simulink model "sampleModel367"  (R2021b)
settings: Solver=VariableStepAuto  StartTime=0.0  StopTime=10.0  RelTol=1e-3
undefined symbols (not defined in the file or in its folder): DiscIntNeverNeededParam
libraries: simulink x15, slpidlib x3
settings Model: Creator=user  LastModifiedBy=user

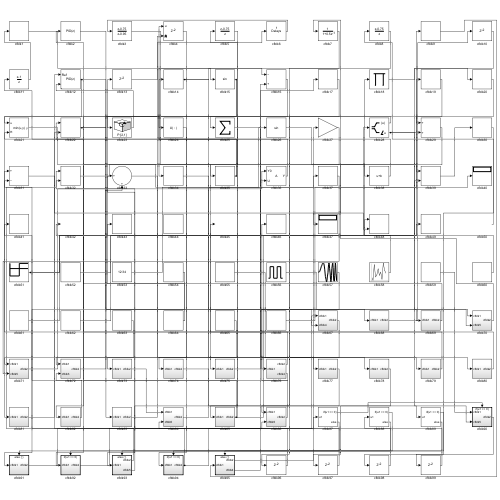
[thumbnail: Simulink's stored preview of the top-level diagram]
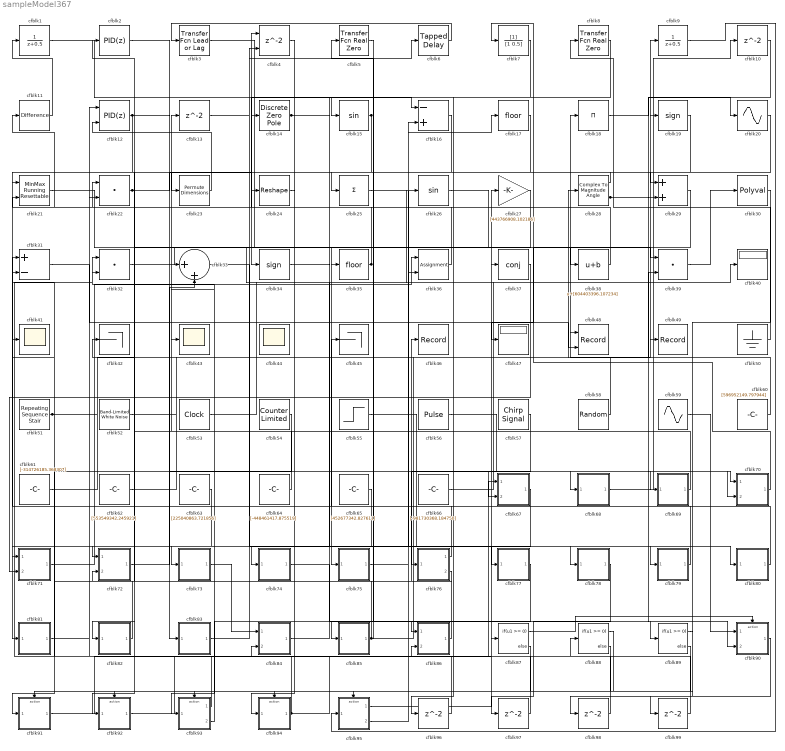
== system sampleModel367 ==
  cfblk1 : DiscreteTransferFcn  SampleTime=1
  cfblk{10,13,96..99} (6 alike) : Delay  SampleTime=1
  cfblk11 : simulink/Discrete/Difference  ICPrevInput=0.0  OutMin=[]  OutMax=[]  OutDataTypeStr=Inherit: Inherit via back propagation  OutDataType=fixdt(1, 16)  OutScaling=2^-10  DoSatur=off
  cfblk12 : slpidlib/PID Controller (2DOF)  Controller=PID  Form=Parallel  TimeDomain=Discrete-time  UseExternalTs=off  SampleTime=1  IntegratorMethod=Forward Euler  FilterMethod=Forward Euler  ControllerParametersSource=internal  P=1  I=1  D=0  UseFilter=on  N=100  b=1  c=1  TunerSelectOption=Transfer Function Based (PID Tuner App)  InitialConditionSource=internal  InitialConditionForIntegrator=0  InitialConditionForFilter=0  DifferentiatorICPrevScaledInput=0  ExternalReset=none  TrackingMode=off  Kt=1  LimitOutput=off  SatLimitsSource=internal  UpperSaturationLimit=inf  LowerSaturationLimit=-inf  LinearizeAsGain=off  AntiWindupMode=none  Kb=1  POutMin=[]  POutMax=[]  IOutMin=[]  IOutMax=[]  DOutMin=[]  DOutMax=[]  NOutMin=[]  NOutMax=[]  bOutMin=[]  bOutMax=[]  cOutMin=[]  cOutMax=[]  SumOutMin=[]  SumOutMax=[]  SaturationOutMin=[]  SaturationOutMax=[]  PParamMin=[]  PParamMax=[]  IParamMin=[]  IParamMax=[]  DParamMin=[]  DParamMax=[]  NParamMin=[]  NParamMax=[]  bParamMin=[]  bParamMax=[]  cParamMin=[]  cParamMax=[]  KbParamMin=[]  KbParamMax=[]  KtParamMin=[]  KtParamMax=[]  KbOutMin=[]  KbOutMax=[]  KtOutMin=[]  KtOutMax=[]  IntegratorOutMin=[]  IntegratorOutMax=[]  FilterOutMin=[]  FilterOutMax=[]  SumI1OutMin=[]  SumI1OutMax=[]  SumI2OutMin=[]  SumI2OutMax=[]  SumI3OutMin=[]  SumI3OutMax=[]  SumI4OutMin=[]  SumI4OutMax=[]  SumDOutMin=[]  SumDOutMax=[]  Sum1OutMin=[]  Sum1OutMax=[]  Sum2OutMin=[]  Sum2OutMax=[]  Sum3OutMin=[]  Sum3OutMax=[]  DifferentiatorOutMin=[]  DifferentiatorOutMax=[]  FilterDiffOutCoefMin=[]  FilterDiffOutCoefMax=[]  ReciprocalOutMin=[]  ReciprocalOutMax=[]  SumDenOutMin=[]  SumDenOutMax=[]  SumNumOutMin=[]  SumNumOutMax=[]  DivideOutMin=[]  DivideOutMax=[]  UdiffTsProdOutMin=[]  UdiffTsProdOutMax=[]  NTsProdOutMin=[]  NTsProdOutMax=[]  UintegralTsProdOutMin=[]  UintegralTsProdOutMax=[]  UngainTsProdOutMin=[]  UngainTsProdOutMax=[]  IntegratorContinuousStateAttributes=''  IntegratorStateMustResolveToSignalObject=off  IntegratorRTWStateStorageClass=Auto  FilterContinuousStateAttributes=''  FilterStateMustResolveToSignalObject=off  FilterRTWStateStorageClass=Auto  ParallelPVariant=InternalParameters  IdealPVariant=Disabled  IVariant=InternalParameters  DVariant=InternalParameters  bVariant=InternalParameters  cVariant=InternalParameters  IntegratorVariant=Discrete  SatVariant=Disabled  AWVariant=Passthrough  PCopyVariant=Disabled  TRVariant=Disabled  FdbkBlocksVariant=Forward  IdealPFdbkVariant=Disabled  SatFdbkVariant=Disabled  DerivativeFilterVariant=ForwardEulerFilter  NVariant=InternalParameters  NCopyVariant=Disabled  FilterICVariant=InternalICsFilter  IntegratorICVariant=InternalICs  ExternalResetVariant=Disabled  TRSumVariant=Passthrough  SumFdbkVariant=Disabled  SumVariant=Sum_PID  TsampFilterVariant=InternalTs  TsampNgainVariant=Passthrough  TsampIntegralVariant=Passthrough  ExternalSaturationOutDataTypeStr=Inherit: Same as second input
      settings: SourceProductBaseCode=SL
  cfblk14 : DiscreteZeroPole  Poles=[0 0.5]  Gain=1
  cfblk15 : Trigonometry
  cfblk16 : Sum  Inputs=-+
  cfblk17 : Rounding
  cfblk18 : Product  Inputs=*
  cfblk19 : Signum
  cfblk2 : slpidlib/PID Controller  Controller=PID  Form=Parallel  TimeDomain=Discrete-time  UseExternalTs=off  SampleTime=1  IntegratorMethod=Forward Euler  FilterMethod=Forward Euler  ControllerParametersSource=internal  P=1  I=1  D=0  UseFilter=on  N=100  TunerSelectOption=Transfer Function Based (PID Tuner App)  InitialConditionSource=internal  InitialConditionForIntegrator=0  InitialConditionForFilter=0  DifferentiatorICPrevScaledInput=0  ExternalReset=none  TrackingMode=off  Kt=1  LimitOutput=off  SatLimitsSource=internal  UpperSaturationLimit=inf  LowerSaturationLimit=-inf  LinearizeAsGain=off  AntiWindupMode=none  Kb=1  POutMin=[]  POutMax=[]  IOutMin=[]  IOutMax=[]  DOutMin=[]  DOutMax=[]  NOutMin=[]  NOutMax=[]  SumOutMin=[]  SumOutMax=[]  SaturationOutMin=[]  SaturationOutMax=[]  PParamMin=[]  PParamMax=[]  IParamMin=[]  IParamMax=[]  DParamMin=[]  DParamMax=[]  NParamMin=[]  NParamMax=[]  KbParamMin=[]  KbParamMax=[]  KtParamMin=[]  KtParamMax=[]  KbOutMin=[]  KbOutMax=[]  KtOutMin=[]  KtOutMax=[]  IntegratorOutMin=[]  IntegratorOutMax=[]  FilterOutMin=[]  FilterOutMax=[]  SumI1OutMin=[]  SumI1OutMax=[]  SumI2OutMin=[]  SumI2OutMax=[]  SumI3OutMin=[]  SumI3OutMax=[]  SumI4OutMin=[]  SumI4OutMax=[]  SumDOutMin=[]  SumDOutMax=[]  DifferentiatorOutMin=[]  DifferentiatorOutMax=[]  FilterDiffOutCoefMin=[]  FilterDiffOutCoefMax=[]  ReciprocalOutMin=[]  ReciprocalOutMax=[]  SumDenOutMin=[]  SumDenOutMax=[]  SumNumOutMin=[]  SumNumOutMax=[]  DivideOutMin=[]  DivideOutMax=[]  UdiffTsProdOutMin=[]  UdiffTsProdOutMax=[]  NTsProdOutMin=[]  NTsProdOutMax=[]  UintegralTsProdOutMin=[]  UintegralTsProdOutMax=[]  UngainTsProdOutMin=[]  UngainTsProdOutMax=[]  IntegratorContinuousStateAttributes=''  IntegratorStateMustResolveToSignalObject=off  IntegratorRTWStateStorageClass=Auto  FilterContinuousStateAttributes=''  FilterStateMustResolveToSignalObject=off  FilterRTWStateStorageClass=Auto  ParallelPVariant=InternalParameters  IdealPVariant=Disabled  IVariant=InternalParameters  DVariant=InternalParameters  IntegratorVariant=Discrete  SatVariant=Disabled  AWVariant=Passthrough  PCopyVariant=Disabled  TRVariant=Disabled  FdbkBlocksVariant=Forward  IdealPFdbkVariant=Disabled  SatFdbkVariant=Disabled  DerivativeFilterVariant=ForwardEulerFilter  NVariant=InternalParameters  NCopyVariant=Disabled  FilterICVariant=InternalICsFilter  IntegratorICVariant=InternalICs  ExternalResetVariant=Disabled  TRSumVariant=Passthrough  SumFdbkVariant=Disabled  SumVariant=Sum_PID  TsampFilterVariant=InternalTs  TsampNgainVariant=Passthrough  TsampIntegralVariant=Passthrough  ExternalSaturationOutDataTypeStr=Inherit: Same as second input
  cfblk20 : Sin  TimeSource=Use external signal  SampleTime=0
  cfblk21 : simulink/Math Operations/MinMax Running Resettable  Function=min  vinit=0.0
  cfblk22 : DotProduct  InputSameDT=on  OutDataTypeStr=Inherit: Inherit via internal rule
  cfblk23 : PermuteDimensions
  cfblk24 : Reshape
  cfblk25 : Sum  Inputs=+
  cfblk26 : Trigonometry
  cfblk27 : Gain  Gain=[443766908.102186]
  cfblk28 : ComplexToMagnitudeAngle
  cfblk29 : Sum
  cfblk3 : simulink/Discrete/Transfer Fcn Lead or Lag  PoleZ=0.95  ZeroZ=0.75  ICPrevOutput=0.0  ICPrevInput=0.0  DoSatur=off
      settings: SourceProductBaseCode=SL
  cfblk30 : Polyval  Coefs=[ +2.081618890e-019, -1.441693666e-014, +4.719686976e-010, -8.536869453e-006, +1.621573104e-001, -8.087801117e+001 ]
  cfblk31 : Sum  Inputs=+-
  cfblk32 : DotProduct  InputSameDT=on  OutDataTypeStr=Inherit: Inherit via internal rule
  cfblk33 : Sum  Inputs=|++
  cfblk34 : Signum
  cfblk35 : Rounding
  cfblk36 : Assignment  DiagnosticForDimensions=Warning  IndexOptions=Index vector (dialog)  Indices=1  OutputSizes=1
  cfblk37 : Math  Operator=conj  SaturateOnIntegerOverflow=on
  cfblk38 : Bias  Bias=[604403396.107234]
  cfblk39 : DotProduct  InputSameDT=on  OutDataTypeStr=Inherit: Inherit via internal rule
  cfblk4 : Delay  ShowEnablePort=on  SampleTime=1
      settings: InputPortMap=u0,e6
  cfblk40 : Display
  cfblk41 : Scope
  cfblk42 : Terminator
  cfblk43 : Scope
  cfblk44 : Scope
      settings: Floating=on
  cfblk45 : Terminator
  cfblk46 : Record  FileSettingsInternal="{\"entries\":[{\"content\":{\"excelSettings\":{\"content\":{},\"type\":\"Streamout.ExcelSettings\"}},\"type\":\"Streamout.FileSettingStorage\",\"uuid\":\"a4817eb2-789e-49c8-9b38-fb696686bad4\"}],\"packageUris\":[\"http://schema.mathworks.com/mf0/streamout_blocks/R2020a\"],\"version\":\"1.0\"}"  SignalsInternal="{\"entries\":[{\"content\":{\"signals\":[{\"content\":{\"blockPath\":[\"sampleModel367/cfblk46\"],\"channel\":[],\"dimensions\":[1],\"domain\":\"sampleModel367/cfblk46\",\"lineColor\":\"#b746ff\",\"plots\":[1],\"port\":1,\"sid\":[\"\"],\"signalID\":15209,\"signalName\":\"cfblk86\"},\"type\":\"RecordBlkView.Signal\",\"uuid\":\"a4bc0313-54ea-4444-9b09-4c15ea739dbc\"}]},\"type\":\"RecordBlkView.InputSignals\",\"uuid\":\"43528cc1-72da-4af5-8b92-5aee9282fc77\"}],\"packageUris\":[\"http://schema.mathworks.com/mf0/streamout_blocks/R2020a\"],\"version\":\"1.0\"}"  VisualizationBindings="{\"sparklinesplugin\":{\"info\":[{\"bindingParametersList\":[],\"subplotID\":1}]}}"
  cfblk47 : Display
  cfblk48 : Record  FileSettingsInternal="{\"entries\":[{\"content\":{\"excelSettings\":{\"content\":{},\"type\":\"Streamout.ExcelSettings\"}},\"type\":\"Streamout.FileSettingStorage\",\"uuid\":\"7f5feb7f-130e-4751-b9c9-40299ce25e98\"}],\"packageUris\":[\"http://schema.mathworks.com/mf0/streamout_blocks/R2020a\"],\"version\":\"1.0\"}"  Layout=[1 1]  SignalsInternal="{\"entries\":[{\"content\":{\"signals\":[{\"content\":{\"blockPath\":[\"sampleModel367/cfblk48\"],\"channel\":[],\"dimensions\":[1],\"domain\":\"sampleModel367/cfblk48\",\"lineColor\":\"#a2142f\",\"plots\":[1],\"port\":1,\"sid\":[\"\"],\"signalID\":15213,\"signalName\":\"cfblk58\"},\"type\":\"RecordBlkView.Signal\",\"uuid\":\"11d3d002-aedb-49d1-ac92-c87df62f412f\"},{\"content\":{\"blockPath\":[\"sampleModel367/cfblk48\"],\"channel\":[],\"dimensions\":[1],\"domain\":\"sampleModel367/cfblk48\",\"lineColor\":\"#139fff\",\"plots\":[1],\"port\":2,\"sid\":[\"\"],\"signalID\":15217,\"signalName\":\"cfblk31\"},\"type\":\"RecordBlkView.Signal\",\"uuid\":\"8ab427da-bc2d-4f3b-aed4-13db8330e9f8\"}]},\"type\":\"RecordBlkView.InputSignals\",\"uuid\":\"18192d45-9ce2-4587-8064-7fff66e14029\"}],\"packageUris\":[\"http://schema.mathworks.com/mf0/streamout_blocks/R2020a\"],\"version\":\"1.0\"}"  VisualizationBindings="{\"xyplotplugin\":{\"info\":[{\"series\":[{\"bindingParametersList\":[{\"parameter\":\"X-Axis\",\"signalID\":15213,\"signalName\":\"cfblk58\"},{\"parameter\":\"Y-Axis\",\"signalID\":15217,\"signalName\":\"cfblk31\"}],\"seriesID\":39746}],\"subplotID\":1}]}}"  CompatibilityTag=XY
  cfblk49 : Record  FileSettingsInternal="{\"entries\":[{\"content\":{\"excelSettings\":{\"content\":{},\"type\":\"Streamout.ExcelSettings\"}},\"type\":\"Streamout.FileSettingStorage\",\"uuid\":\"f483f2fa-4d2d-4028-bd3b-ca284f8ff664\"}],\"packageUris\":[\"http://schema.mathworks.com/mf0/streamout_blocks/R2020a\"],\"version\":\"1.0\"}"  SignalsInternal="{\"entries\":[{\"content\":{\"signals\":[{\"content\":{\"blockPath\":[\"sampleModel367/cfblk49\"],\"channel\":[],\"dimensions\":[1],\"domain\":\"sampleModel367/cfblk49\",\"lineColor\":\"#fe330a\",\"plots\":[1],\"port\":1,\"sid\":[\"\"],\"signalID\":15221,\"signalName\":\"cfblk52\"},\"type\":\"RecordBlkView.Signal\",\"uuid\":\"1644548f-0715-4922-8539-540d67eabf0f\"}]},\"type\":\"RecordBlkView.InputSignals\",\"uuid\":\"b89c8940-25df-486a-b77a-2b62a827f3dc\"}],\"packageUris\":[\"http://schema.mathworks.com/mf0/streamout_blocks/R2020a\"],\"version\":\"1.0\"}"  VisualizationBindings="{\"sparklinesplugin\":{\"info\":[{\"bindingParametersList\":[],\"subplotID\":1}]}}"
  cfblk5 : simulink/Discrete/Transfer Fcn Real Zero  ZeroZ=0.75  ICPrevInput=0.0  DoSatur=off
      settings: SourceProductBaseCode=SL
  cfblk50 : Ground
  cfblk51 : simulink/Sources/Repeating Sequence Stair  OutValues=[-738715956.352001, 505960308.450328]  tsamp=-1  OutMin=[]  OutMax=[]  OutDataTypeStr=double  OutputDataTypeScalingMode=double  OutDataType=fixdt(0,8)  ConRadixGroup=Best Precision: Vector-wise  OutScaling=2^-12
  cfblk52 : simulink/Sources/Band-Limited White Noise  Cov=[2265399686.843978]  Ts=0.1  seed=[1401870864.000000]
  cfblk53 : DigitalClock
  cfblk54 : simulink/Sources/Counter Limited  uplimit=[456.000000]  tsamp=-1
  cfblk55 : Step  Time=[22.000000]  Before=[489707741.250540]  After=[-608440485.162170]  SampleTime=0
  cfblk56 : DiscretePulseGenerator  PulseType=Time based  Amplitude=[-325333770.550058]  Period=[52379731.068444]  PulseWidth=5  PhaseDelay=[5.000000]
  cfblk57 : simulink/Sources/Chirp Signal  f1=[608529907.100524]  T=[-869781854.255579]  f2=[19229579.544887]
  cfblk58 : UniformRandomNumber  Minimum=[-2920603803.770856]  Maximum=[4155902008.419292]  Seed=[92260786.000000]  SampleTime=0.1
  cfblk59 : Sin  Amplitude=[-802528330.352134]  Bias=[221052737.298731]  SampleTime=0
  cfblk6 : simulink/Discrete/Tapped Delay  vinit=0.0  samptime=-1  NumDelays=1  DelayOrder=Oldest  includeCurrent=off
  cfblk60 : Constant  Value=[596952149.797944]  SampleTime=1
  cfblk61 : Constant  Value=[-314726185.368307]  SampleTime=1
  cfblk62 : Constant  Value=[553549342.245921]  SampleTime=1
  cfblk63 : Constant  Value=[225040863.721856]  SampleTime=1
  cfblk64 : Constant  Value=[-448461417.875519]  SampleTime=1
  cfblk65 : Constant  Value=[452677342.827611]  SampleTime=1
  cfblk66 : Constant  Value=[-981730368.184750]  SampleTime=1
  cfblk67 : Subsystem
  cfblk68 : Subsystem
  cfblk69 : Subsystem
  cfblk7 : DiscreteFilter  SampleTime=1
  cfblk70 : Subsystem
  cfblk71 : Subsystem
  cfblk72 : Subsystem
  cfblk73 : Subsystem
  cfblk74 : Subsystem
  cfblk75 : Subsystem
  cfblk76 : Subsystem
  cfblk77 : Subsystem
  cfblk78 : Subsystem
  cfblk79 : Subsystem
  cfblk8 : simulink/Discrete/Transfer Fcn Real Zero  ZeroZ=0.75  ICPrevInput=0.0  DoSatur=off
      settings: SourceProductBaseCode=SL
  cfblk80 : Subsystem
  cfblk81 : Subsystem
  cfblk82 : Subsystem
  cfblk83 : Subsystem
  cfblk84 : Subsystem
  cfblk85 : Subsystem
  cfblk86 : Subsystem
  cfblk87 : If  IfExpression=u1 >= 0  SampleTime=1
  cfblk88 : If  IfExpression=u1 >= 0  SampleTime=1
  cfblk89 : If  IfExpression=u1 >= 0  SampleTime=1
  cfblk9 : DiscreteTransferFcn  SampleTime=1
  cfblk90 : Subsystem  TreatAsAtomicUnit=on
  cfblk91 : Subsystem  TreatAsAtomicUnit=on
  cfblk92 : Subsystem  TreatAsAtomicUnit=on
  cfblk93 : Subsystem  TreatAsAtomicUnit=on
  cfblk94 : Subsystem  TreatAsAtomicUnit=on
  cfblk95 : Subsystem  TreatAsAtomicUnit=on
  wires:
  cfblk71/1(cfblk2) -> cfblk36/1
  cfblk7/1 -> cfblk34/1
  cfblk60/1 -> cfblk18/1
  cfblk93/1(cfblk2) -> cfblk32/1
  cfblk59/1 -> cfblk90/1(cfblk1)
  cfblk32/1 -> cfblk26/1
  cfblk73/1(cfblk2) -> cfblk84/1(cfblk1)
  cfblk95/1(cfblk2) -> cfblk27/1
  cfblk27/1 -> cfblk72/1(cfblk1)
  cfblk1/1 -> cfblk15/1
  cfblk70/1(cfblk2) -> cfblk7/1
  cfblk68/1(cfblk2) -> cfblk10/1
  cfblk86/1(cfblk2) -> cfblk46/1
  cfblk51/1 -> cfblk13/1, cfblk39/2
  cfblk4/1 -> cfblk74/1(cfblk1)
  cfblk25/1 -> cfblk79/1(cfblk1)
  cfblk85/1(cfblk2) -> cfblk9/1, cfblk42/1, cfblk5/1
  cfblk14/1 -> cfblk16/1, cfblk78/1(cfblk1)
  cfblk61/1 -> cfblk16/2
  cfblk39/1 -> cfblk30/1
  cfblk23/1 -> cfblk12/2
  cfblk28/1 -> cfblk25/1
  cfblk93/2(cfblk5) -> cfblk32/2
  cfblk21/1 -> cfblk75/1(cfblk1)
  cfblk56/1 -> cfblk68/1(cfblk1)
  cfblk58/1 -> cfblk48/1
  cfblk11/1 -> cfblk1/1
  cfblk53/1 -> cfblk19/1
  cfblk31/1 -> cfblk48/2
  cfblk12/1 -> cfblk81/1(cfblk1), cfblk70/2(cfblk5)
  cfblk69/1(cfblk2) -> cfblk2/1
  cfblk80/1(cfblk2) -> cfblk31/1
  cfblk66/1 -> cfblk40/1
  cfblk57/1 -> cfblk76/1(cfblk1)
  cfblk79/1(cfblk2) -> cfblk45/1
  cfblk19/1 -> cfblk85/1(cfblk1)
  cfblk2/1 -> cfblk83/1(cfblk1)
  cfblk5/1 -> cfblk35/1
  cfblk8/1 -> cfblk86/1(cfblk1)
  cfblk54/1 -> cfblk91/1(cfblk1)
  cfblk26/1 -> cfblk39/1
  cfblk24/1 -> cfblk94/1(cfblk1)
  cfblk67/1(cfblk2) -> cfblk73/1(cfblk1)
  cfblk33/1 -> cfblk77/1(cfblk1)
  cfblk16/1 -> cfblk21/1
  cfblk76/1(cfblk2) -> cfblk22/1
  cfblk9/1 -> cfblk95/1(cfblk1)
  cfblk50/1 -> cfblk8/1
  cfblk81/1(cfblk2) -> cfblk22/2
  cfblk64/1 -> cfblk43/1
  cfblk55/1 -> cfblk80/1(cfblk1)
  cfblk52/1 -> cfblk49/1
  cfblk84/1(cfblk2) -> cfblk37/1
  cfblk6/1 -> cfblk3/1
  cfblk75/1(cfblk2) -> cfblk17/1
  cfblk63/1 -> cfblk82/1(cfblk1)
  cfblk18/1 -> cfblk20/1
  cfblk62/1 -> cfblk28/1
  cfblk38/1 -> cfblk4/1
  cfblk15/1 -> cfblk23/1, cfblk92/1(cfblk1)
  cfblk20/1 -> cfblk29/1
  cfblk74/1(cfblk2) -> cfblk89/1
  cfblk3/1 -> cfblk38/1
  cfblk92/1(cfblk2) -> cfblk87/1
  cfblk65/1 -> cfblk71/1(cfblk1)
  cfblk36/1 -> cfblk14/1
  cfblk29/1 -> cfblk47/1
  cfblk10/1 -> cfblk29/2
  cfblk28/2 -> cfblk90/2(cfblk5), cfblk70/1(cfblk1)
  cfblk91/1(cfblk2) -> cfblk67/1(cfblk1)
  cfblk34/1 -> cfblk69/1(cfblk1)
  cfblk76/2(cfblk4) -> cfblk72/2(cfblk3)
  cfblk37/1 -> cfblk71/2(cfblk5)
  cfblk22/1 -> cfblk67/2(cfblk4), cfblk24/1
  cfblk94/1(cfblk2) -> cfblk31/2, cfblk86/2(cfblk5)
  cfblk82/1(cfblk2) -> cfblk41/1
  cfblk77/1(cfblk2) -> cfblk93/1(cfblk1)
  cfblk35/1 -> cfblk21/2, cfblk11/1
  cfblk13/1 -> cfblk6/1
  cfblk83/1(cfblk2) -> cfblk4/2
  cfblk72/1(cfblk2) -> cfblk33/2
  cfblk95/2(cfblk4) -> cfblk36/2
  cfblk87/1 -> cfblk90/Action
  cfblk87/2 -> cfblk91/Action
  cfblk88/1 -> cfblk92/Action
  cfblk88/2 -> cfblk93/Action
  cfblk89/1 -> cfblk94/Action
  cfblk89/2 -> cfblk95/Action
  cfblk17/1 -> cfblk96/1
  cfblk96/1 -> cfblk12/1
  cfblk78/1(cfblk2) -> cfblk97/1
  cfblk97/1 -> cfblk84/2(cfblk5)
  cfblk90/1(cfblk2) -> cfblk98/1
  cfblk98/1 -> cfblk33/1
  cfblk30/1 -> cfblk99/1
  cfblk99/1 -> cfblk88/1

== system sampleModel367/cfblk67 ==
  cfblk1 : Inport
  cfblk4 : Inport  Port=2
  cfblk3 : Constant  Value=[791161119.661212]  SampleTime=1
  cfblk2 : Outport
  wires:
  cfblk3/1 -> cfblk2/1

== system sampleModel367/cfblk68 ==
  cfblk1 : Inport
  cfblk3 : slpidlib/PID Controller (2DOF)  Controller=PID  Form=Parallel  TimeDomain=Discrete-time  UseExternalTs=off  SampleTime=1  IntegratorMethod=Forward Euler  FilterMethod=Forward Euler  ControllerParametersSource=internal  P=1  I=1  D=0  UseFilter=on  N=100  b=1  c=1  TunerSelectOption=Transfer Function Based (PID Tuner App)  InitialConditionSource=internal  InitialConditionForIntegrator=0  InitialConditionForFilter=0  DifferentiatorICPrevScaledInput=0  ExternalReset=none  TrackingMode=off  Kt=1  LimitOutput=off  SatLimitsSource=internal  UpperSaturationLimit=inf  LowerSaturationLimit=-inf  LinearizeAsGain=off  AntiWindupMode=none  Kb=1  POutMin=[]  POutMax=[]  IOutMin=[]  IOutMax=[]  DOutMin=[]  DOutMax=[]  NOutMin=[]  NOutMax=[]  bOutMin=[]  bOutMax=[]  cOutMin=[]  cOutMax=[]  SumOutMin=[]  SumOutMax=[]  SaturationOutMin=[]  SaturationOutMax=[]  PParamMin=[]  PParamMax=[]  IParamMin=[]  IParamMax=[]  DParamMin=[]  DParamMax=[]  NParamMin=[]  NParamMax=[]  bParamMin=[]  bParamMax=[]  cParamMin=[]  cParamMax=[]  KbParamMin=[]  KbParamMax=[]  KtParamMin=[]  KtParamMax=[]  KbOutMin=[]  KbOutMax=[]  KtOutMin=[]  KtOutMax=[]  IntegratorOutMin=[]  IntegratorOutMax=[]  FilterOutMin=[]  FilterOutMax=[]  SumI1OutMin=[]  SumI1OutMax=[]  SumI2OutMin=[]  SumI2OutMax=[]  SumI3OutMin=[]  SumI3OutMax=[]  SumI4OutMin=[]  SumI4OutMax=[]  SumDOutMin=[]  SumDOutMax=[]  Sum1OutMin=[]  Sum1OutMax=[]  Sum2OutMin=[]  Sum2OutMax=[]  Sum3OutMin=[]  Sum3OutMax=[]  DifferentiatorOutMin=[]  DifferentiatorOutMax=[]  FilterDiffOutCoefMin=[]  FilterDiffOutCoefMax=[]  ReciprocalOutMin=[]  ReciprocalOutMax=[]  SumDenOutMin=[]  SumDenOutMax=[]  SumNumOutMin=[]  SumNumOutMax=[]  DivideOutMin=[]  DivideOutMax=[]  UdiffTsProdOutMin=[]  UdiffTsProdOutMax=[]  NTsProdOutMin=[]  NTsProdOutMax=[]  UintegralTsProdOutMin=[]  UintegralTsProdOutMax=[]  UngainTsProdOutMin=[]  UngainTsProdOutMax=[]  IntegratorContinuousStateAttributes=''  IntegratorStateMustResolveToSignalObject=off  IntegratorRTWStateStorageClass=Auto  FilterContinuousStateAttributes=''  FilterStateMustResolveToSignalObject=off  FilterRTWStateStorageClass=Auto  ParallelPVariant=InternalParameters  IdealPVariant=Disabled  IVariant=InternalParameters  DVariant=InternalParameters  bVariant=InternalParameters  cVariant=InternalParameters  IntegratorVariant=Discrete  SatVariant=Disabled  AWVariant=Passthrough  PCopyVariant=Disabled  TRVariant=Disabled  FdbkBlocksVariant=Forward  IdealPFdbkVariant=Disabled  SatFdbkVariant=Disabled  DerivativeFilterVariant=ForwardEulerFilter  NVariant=InternalParameters  NCopyVariant=Disabled  FilterICVariant=InternalICsFilter  IntegratorICVariant=InternalICs  ExternalResetVariant=Disabled  TRSumVariant=Passthrough  SumFdbkVariant=Disabled  SumVariant=Sum_PID  TsampFilterVariant=InternalTs  TsampNgainVariant=Passthrough  TsampIntegralVariant=Passthrough  ExternalSaturationOutDataTypeStr=Inherit: Same as second input
      settings: SourceProductBaseCode=SL
  cfblk2 : Outport
  wires:
  cfblk1/1 -> cfblk2/1, cfblk3/1, cfblk3/2

== system sampleModel367/cfblk69 ==
  cfblk1 : Inport
  cfblk3 : DiscreteFir  SampleTime=1
  cfblk2 : Outport
  wires:
  cfblk1/1 -> cfblk3/1
  cfblk3/1 -> cfblk2/1

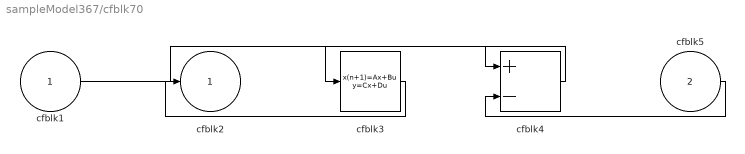
== system sampleModel367/cfblk70 ==
  cfblk1 : Inport
  cfblk5 : Inport  Port=2
  cfblk3 : DiscreteStateSpace
  cfblk4 : Sum  Inputs=+-
  cfblk2 : Outport
  wires:
  cfblk1/1 -> cfblk4/1
  cfblk5/1 -> cfblk4/2
  cfblk4/1 -> cfblk3/1
  cfblk3/1 -> cfblk2/1

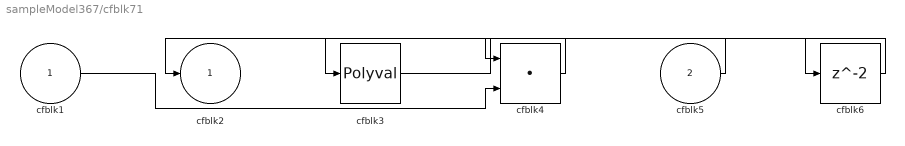
== system sampleModel367/cfblk71 ==
  cfblk1 : Inport
  cfblk5 : Inport  Port=2
  cfblk3 : Polyval  Coefs=[ +2.081618890e-019, -1.441693666e-014, +4.719686976e-010, -8.536869453e-006, +1.621573104e-001, -8.087801117e+001 ]
  cfblk4 : DotProduct  InputSameDT=on  OutDataTypeStr=Inherit: Inherit via internal rule
  cfblk6 : Delay  SampleTime=1
  cfblk2 : Outport
  wires:
  cfblk5/1 -> cfblk2/1
  cfblk1/1 -> cfblk4/2
  cfblk4/1 -> cfblk3/1
  cfblk3/1 -> cfblk6/1
  cfblk6/1 -> cfblk4/1

== system sampleModel367/cfblk72 ==
  cfblk1 : Inport
  cfblk3 : Inport  Port=2
  cfblk2 : Outport
  wires:
  cfblk3/1 -> cfblk2/1

== system sampleModel367/cfblk73 ==
  cfblk1 : Inport
  cfblk3 : Constant  Value=[161644396.941690]  SampleTime=1
  cfblk2 : Outport
  wires:
  cfblk1/1 -> cfblk2/1

== system sampleModel367/cfblk74 ==
  cfblk1 : Inport
  cfblk3 : ComplexToRealImag
  cfblk2 : Outport
  wires:
  cfblk1/1 -> cfblk3/1
  cfblk3/1 -> cfblk2/1

== system sampleModel367/cfblk75 ==
  cfblk1 : Inport
  cfblk3 : Sum  Inputs=+
  cfblk2 : Outport
  wires:
  cfblk1/1 -> cfblk2/1, cfblk3/1

== system sampleModel367/cfblk76 ==
  cfblk1 : Inport
  cfblk3 : Delay  DelayLengthSource=Input port  SampleTime=1
      settings: InputPortMap=u0,p1
  cfblk2 : Outport
  cfblk4 : Outport  Port=2
  wires:
  cfblk3/1 -> cfblk4/1
  cfblk1/1 -> cfblk2/1, cfblk3/1, cfblk3/2

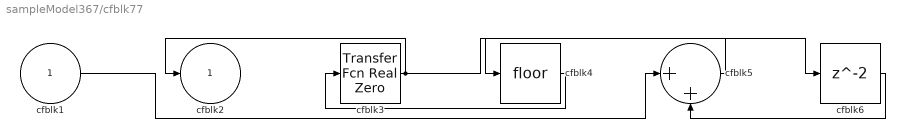
== system sampleModel367/cfblk77 ==
  cfblk1 : Inport
  cfblk3 : simulink/Discrete/Transfer Fcn Real Zero  ZeroZ=0.75  ICPrevInput=0.0  DoSatur=off
      settings: SourceProductBaseCode=SL
  cfblk4 : Rounding
  cfblk5 : Sum  Inputs=|++
  cfblk6 : Delay  SampleTime=1
  cfblk2 : Outport
  wires:
  cfblk3/1 -> cfblk2/1, cfblk6/1
  cfblk5/1 -> cfblk4/1
  cfblk4/1 -> cfblk3/1
  cfblk1/1 -> cfblk5/1
  cfblk6/1 -> cfblk5/2

== system sampleModel367/cfblk78 ==
  cfblk1 : Inport
  cfblk3 : DotProduct  InputSameDT=on  OutDataTypeStr=Inherit: Inherit via internal rule
  cfblk2 : Outport
  wires:
  cfblk1/1 -> cfblk2/1, cfblk3/1, cfblk3/2

== system sampleModel367/cfblk79 ==
  cfblk1 : Inport
  cfblk3 : DotProduct  InputSameDT=on  OutDataTypeStr=Inherit: Inherit via internal rule
  cfblk2 : Outport
  wires:
  cfblk3/1 -> cfblk2/1
  cfblk1/1 -> cfblk3/1, cfblk3/2

== system sampleModel367/cfblk80 ==
  cfblk1 : Inport
  cfblk3 : DiscreteZeroPole  Poles=[0 0.5]  Gain=1
  cfblk2 : Outport
  wires:
  cfblk1/1 -> cfblk3/1
  cfblk3/1 -> cfblk2/1

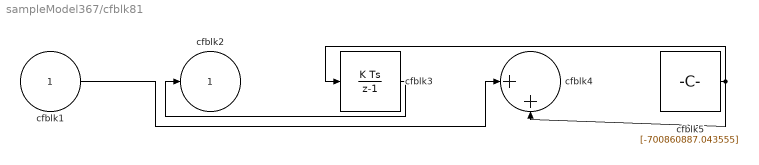
== system sampleModel367/cfblk81 ==
  cfblk1 : Inport
  cfblk3 : DiscreteIntegrator  ICPrevOutput=DiscIntNeverNeededParam  ICPrevScaledInput=DiscIntNeverNeededParam
  cfblk4 : Sum  Inputs=|++
  cfblk5 : Constant  Value=[-700860887.043555]  SampleTime=1
  cfblk2 : Outport
  wires:
  cfblk5/1 -> cfblk3/1, cfblk4/2
  cfblk3/1 -> cfblk2/1
  cfblk1/1 -> cfblk4/1

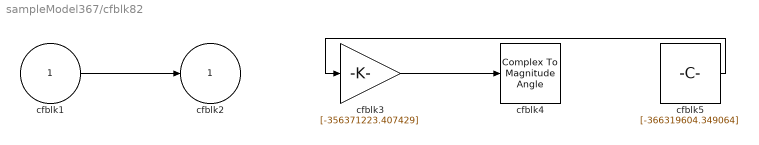
== system sampleModel367/cfblk82 ==
  cfblk1 : Inport
  cfblk3 : Gain  Gain=[-356371223.407429]
  cfblk4 : ComplexToMagnitudeAngle
  cfblk5 : Constant  Value=[-366319604.349064]  SampleTime=1
  cfblk2 : Outport
  wires:
  cfblk1/1 -> cfblk2/1
  cfblk5/1 -> cfblk3/1
  cfblk3/1 -> cfblk4/1

== system sampleModel367/cfblk83 ==
  cfblk1 : Inport
  cfblk3 : simulink/Discrete/Transfer Fcn Lead or Lag  PoleZ=0.95  ZeroZ=0.75  ICPrevOutput=0.0  ICPrevInput=0.0  DoSatur=off
      settings: SourceProductBaseCode=SL
  cfblk4 : simulink/Math Operations/MinMax Running Resettable  Function=min  vinit=0.0
  cfblk2 : Outport
  wires:
  cfblk4/1 -> cfblk2/1
  cfblk1/1 -> cfblk3/1, cfblk4/2
  cfblk3/1 -> cfblk4/1

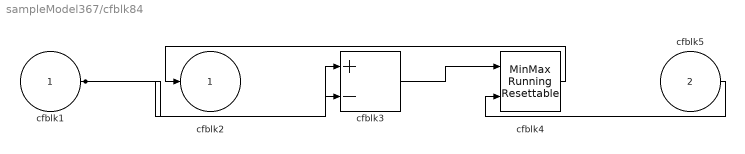
== system sampleModel367/cfblk84 ==
  cfblk1 : Inport
  cfblk5 : Inport  Port=2
  cfblk3 : Sum  Inputs=+-
  cfblk4 : simulink/Math Operations/MinMax Running Resettable  Function=min  vinit=0.0
  cfblk2 : Outport
  wires:
  cfblk3/1 -> cfblk4/1
  cfblk5/1 -> cfblk4/2
  cfblk4/1 -> cfblk2/1
  cfblk1/1 -> cfblk3/1, cfblk3/2

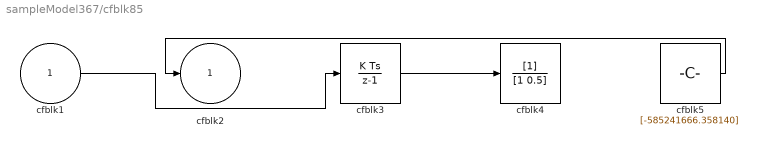
== system sampleModel367/cfblk85 ==
  cfblk1 : Inport
  cfblk3 : DiscreteIntegrator  ICPrevOutput=DiscIntNeverNeededParam  ICPrevScaledInput=DiscIntNeverNeededParam
  cfblk4 : DiscreteFilter  SampleTime=1
  cfblk5 : Constant  Value=[-585241666.358140]  SampleTime=1
  cfblk2 : Outport
  wires:
  cfblk5/1 -> cfblk2/1
  cfblk1/1 -> cfblk3/1
  cfblk3/1 -> cfblk4/1

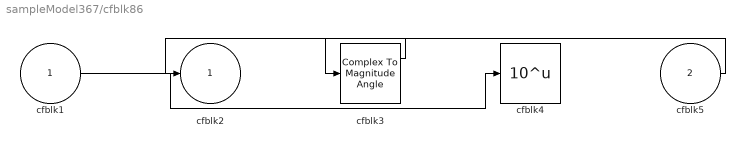
== system sampleModel367/cfblk86 ==
  cfblk1 : Inport
  cfblk5 : Inport  Port=2
  cfblk3 : ComplexToMagnitudeAngle
  cfblk4 : Math  Operator=10^u  SaturateOnIntegerOverflow=on
  cfblk2 : Outport
  wires:
  cfblk5/1 -> cfblk3/1
  cfblk1/1 -> cfblk4/1
  cfblk3/1 -> cfblk2/1

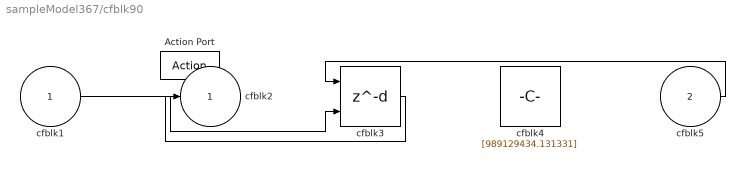
== system sampleModel367/cfblk90 ==
  cfblk1 : Inport
  cfblk5 : Inport  Port=2
  Action Port : ActionPort  ActionPortLabel=if(u1 >= 0)
  cfblk3 : Delay  DelayLengthSource=Input port
      settings: InputPortMap=u0,p1
  cfblk4 : Constant  Value=[989129434.131331]  SampleTime=1
  cfblk2 : Outport
  wires:
  cfblk5/1 -> cfblk3/1
  cfblk1/1 -> cfblk3/2
  cfblk3/1 -> cfblk2/1

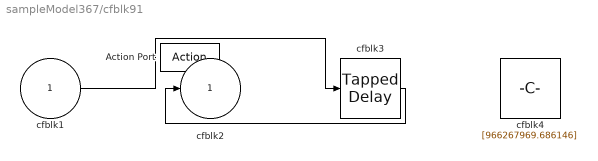
== system sampleModel367/cfblk91 ==
  cfblk1 : Inport
  Action Port : ActionPort  ActionPortLabel=else
  cfblk3 : simulink/Discrete/Tapped Delay  vinit=0.0  samptime=-1  NumDelays=1  DelayOrder=Oldest  includeCurrent=off
  cfblk4 : Constant  Value=[966267969.686146]  SampleTime=1
  cfblk2 : Outport
  wires:
  cfblk3/1 -> cfblk2/1
  cfblk1/1 -> cfblk3/1

== system sampleModel367/cfblk92 ==
  cfblk1 : Inport
  Action Port : ActionPort  ActionPortLabel=if(u1 >= 0)
  cfblk3 : Rounding
  cfblk2 : Outport
  wires:
  cfblk1/1 -> cfblk3/1
  cfblk3/1 -> cfblk2/1

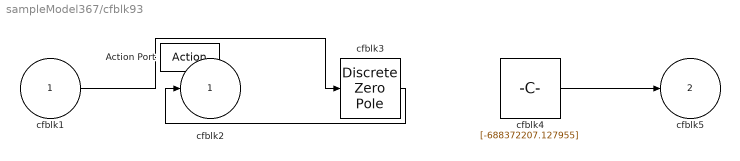
== system sampleModel367/cfblk93 ==
  cfblk1 : Inport
  Action Port : ActionPort  ActionPortLabel=else
  cfblk3 : DiscreteZeroPole  Poles=[0 0.5]  Gain=1  SampleTime=-1
  cfblk4 : Constant  Value=[-688372207.127955]  SampleTime=1
  cfblk2 : Outport
  cfblk5 : Outport  Port=2
  wires:
  cfblk3/1 -> cfblk2/1
  cfblk1/1 -> cfblk3/1
  cfblk4/1 -> cfblk5/1

== system sampleModel367/cfblk94 ==
  cfblk1 : Inport
  Action Port : ActionPort  ActionPortLabel=if(u1 >= 0)
  cfblk3 : UnaryMinus
  cfblk2 : Outport
  wires:
  cfblk3/1 -> cfblk2/1
  cfblk1/1 -> cfblk3/1

== system sampleModel367/cfblk95 ==
  cfblk1 : Inport
  Action Port : ActionPort  ActionPortLabel=else
  cfblk3 : UnitDelay  SampleTime=-1  HasFrameUpgradeWarning=on
  cfblk2 : Outport
  cfblk4 : Outport  Port=2
  wires:
  cfblk1/1 -> cfblk4/1, cfblk3/1
  cfblk3/1 -> cfblk2/1
